simulink model "miniproject"  (R2015a)
settings: Solver=ode45  StartTime=0.0  StopTime=10.0  RelTol=1e-3
libraries: powerlib x6, simulink x3, powerlib_meascontrol x1
settings Model: Creator=karan  LastModifiedBy=karan

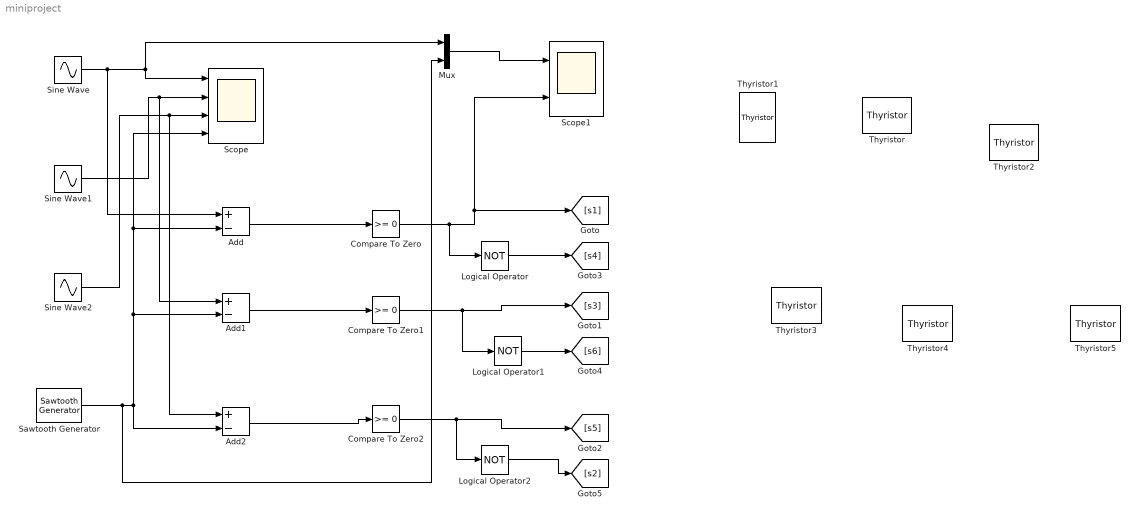
== system miniproject ==
  Add : Sum  Inputs=+-
  Add1 : Sum  Inputs=+-
  Add2 : Sum  Inputs=+-
  Compare To Zero : simulink/Logic and Bit Operations/Compare To Zero  relop=>=  OutDataTypeStr=boolean
  Compare To Zero1 : simulink/Logic and Bit Operations/Compare To Zero  relop=>=  OutDataTypeStr=boolean
  Compare To Zero2 : simulink/Logic and Bit Operations/Compare To Zero  relop=>=  OutDataTypeStr=boolean
  Logical Operator : Logic  Operator=NOT  AllPortsSameDT=off  OutDataTypeStr=boolean
  Logical Operator1 : Logic  Operator=NOT  AllPortsSameDT=off  OutDataTypeStr=boolean
  Logical Operator2 : Logic  Operator=NOT  AllPortsSameDT=off  OutDataTypeStr=boolean
  Mux : Mux  Inputs=2
  Sawtooth Generator : powerlib_meascontrol/Pulse & Signal Generators/Sawtooth Generator  Freq=1e3  Phase=180  Ts=0
  Scope : Scope  NumInputPorts=4
      settings: TimeRange=0.06606551724138576  YMin=-1~-1~-0.7857142857142856~-1  YMax=1~1~-0.7222222222222214~1
  Scope1 : Scope  NumInputPorts=2
      settings: TimeRange=0.06606551724138576  YMin=-1~-5  YMax=1~5
  Sine Wave : Sin  Frequency=2*pi*50  SampleTime=0
  Sine Wave1 : Sin  Frequency=2*pi*50  Phase=2*pi/3  SampleTime=0
  Sine Wave2 : Sin  Frequency=2*pi*50  Phase=-2*pi/3  SampleTime=0
  Thyristor{,1..5} (6 alike) : powerlib/Power Electronics/Thyristor  Ron=0.001  Lon=0  Vf=0.8  IC=0  Rs=500  Cs=250e-9  Measurements=on
  wires:
  Sine Wave/1 -> Add/1, Scope/1, Mux/1
  Sine Wave1/1 -> Add1/1, Scope/2
  Sine Wave2/1 -> Add2/1, Scope/3
  Sawtooth Generator/1 -> Mux/2, Add/2, Scope/4, Add1/2, Add2/2
  Add/1 -> Compare To Zero/1
  Add1/1 -> Compare To Zero1/1
  Add2/1 -> Compare To Zero2/1
  Compare To Zero/1 -> Logical Operator/1, [s1], Scope1/2
  Mux/1 -> Scope1/1
  Compare To Zero1/1 -> Logical Operator1/1, [s3]
  Compare To Zero2/1 -> Logical Operator2/1, [s5]
  Logical Operator/1 -> [s4]
  Logical Operator1/1 -> [s6]
  Logical Operator2/1 -> [s2]
